simulink model "Assignment7"  (R2021a)
settings: Solver=FixedStepDiscrete  StartTime=0.0  StopTime=20  RelTol=1e-3
settings Model: Creator=OmarMedhat  LastModifiedBy=OmarMedhat
settings OptimizationCC: DefaultParameterBehavior=Inlined  EnhancedBackFolding=on  PassReuseOutputArgsAs=Individual arguments  ZeroExternalMemoryAtStartup=off  ZeroInternalMemoryAtStartup=off  OptimizeBlockOrder=speed  DifferentSizesBufferReuse=on  OptimizationCustomize=off  EfficientTunableParamExpr=on
settings DebuggingCC: ParameterTunabilityLossMsg=error
settings SFSimCC: MATLABDynamicMemAlloc=off
settings RTWCC: SystemTargetFile=ert.tlc  GenCodeOnly=on  TemplateMakefile=ert_default_tmf  GenerateReport=on  IncludeHyperlinkInReport=on  LaunchReport=on  GenerateTraceInfo=on
settings CodeAppCC: ForceParamTrailComments=on  IgnoreCustomStorageClasses=off  OperatorAnnotations=on  SimulinkDataObjDesc=on  SFDataObjDesc=on  InsertBlockDesc=on
settings ERTTargetCC: TargetLangStandard=C99 (ISO)  GenerateSampleERTMain=on  InlinedParameterPlacement=NonHierarchical  ERTCustomFileTemplate=example_file_process.tlc

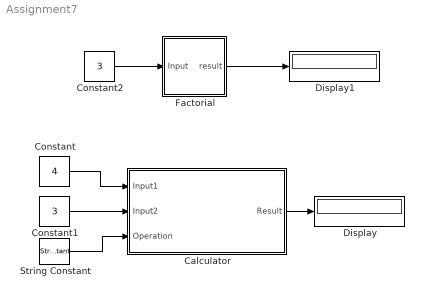
== system Assignment7 ==
  Calculator : Stateflow chart  TreatAsAtomicUnit=on
  Constant : Constant  Value=4  OutDataTypeStr=uint16
  Constant1 : Constant  Value=3  OutDataTypeStr=uint16
  Constant2 : Constant  Value=3  OutDataTypeStr=uint16
  Display : Display
  Display1 : Display
  Factorial : Stateflow chart  TreatAsAtomicUnit=on
  String Constant : StringConstant  String='*'
  wires:
  Calculator/1(Result) -> Display/1
  Constant/1 -> Calculator/1(Input1)
  Constant1/1 -> Calculator/2(Input2)
  String Constant/1 -> Calculator/3(Operation)
  Constant2/1 -> Factorial/1(Input)
  Factorial/1(result) -> Display1/1

== stateflow chart Assignment7/Factorial ==
  (default) -> (junction 9) : /* Factorial */
  (junction 9) -> (junction 11)
  (junction 11) -> (junction 10) [order 1] : [index<=Input]
  (junction 12) -> (junction 11)
  (junction 10) -> (junction 12) : {result=result*index;
      |  index++ ; }
  (junction 11) -> (junction 13) [order 2]
  data: Input input uint16; result output uint16 =1; index local uint16 =1

== stateflow chart Assignment7/Calculator ==
  state Calculator(Input1,Input2) [function]
    (default) -> (junction 165) : % OperationSwitch
    (junction 165) -> (junction 169) [order 1] : [Operation == '+']
    (junction 165) -> (junction 168) [order 2]
    (junction 169) -> (junction 173) : {Result=Input1 + Input2 ;}
    (junction 173) -> (junction 166)
    (junction 166) -> (junction 171)
    (junction 168) -> (junction 167) [order 1] : [Operation == '-']
    (junction 168) -> (junction 172) [order 2]
    (junction 167) -> (junction 170) : {Result=Input1 - Input2;}
    (junction 170) -> (junction 171)
    (junction 171) -> (junction 183)
    (junction 172) -> (junction 179) [order 1] : [Operation == '*']
    (junction 172) -> (junction 176) [order 2]
    (junction 179) -> (junction 175) : {Result=Input1 * Input2 ;}
    (junction 175) -> (junction 183)
    (junction 183) -> (junction 180)
    (junction 176) -> (junction 178) [order 1] : [Operation == '/']
    (junction 176) -> (junction 177) [order 2]
    (junction 178) -> (junction 174) : {Result=Input1 / Input2 ;}
    (junction 174) -> (junction 180)
    (junction 180) -> (junction 181)
    (junction 181) -> (junction 177)
    (junction 177) -> (junction 182)
  note: Do not put any code along
      | the transitions that run
      | down the right side!
  (default) -> (junction 184) : {Calculator(Input1,Input2);}
  data: Input1 function_input double; Input2 function_input double; Input1 input uint16; Input2 input uint16; Result output uint16; Operation input
